simulink model "Tank_Backsteping_Adaptative_TIF"  (R2025b)
settings: Solver=ode45  StartTime=0.0  StopTime=250  RelTol=1e-3
model workspace (MAT data in the model file):
  Vp = Simulink.Parameter
  Vp.Complexity = 'real'
  Vp.Dimensions = [0 0]
  Vp.DataType = 'auto'
settings Model: Creator=juerg
settings DataIOCC: ReturnWorkspaceOutputs=off

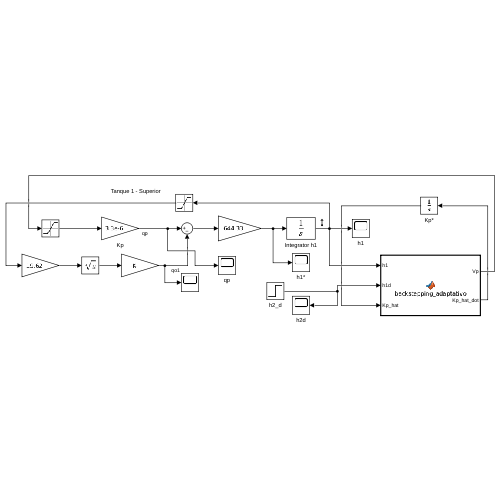
[thumbnail: Simulink's stored preview of the top-level diagram]
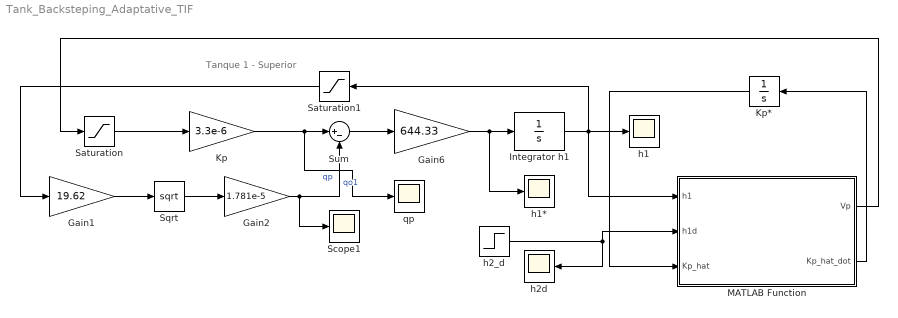
== system Tank_Backsteping_Adaptative_TIF ==
  note: Tanque 1 - Superior
  Gain1 : Gain  Gain=19.62
  Gain2 : Gain  Gain=1.781e-5
  Gain6 : Gain  Gain=644.33
  Integrator h1 : Integrator
  Kp : Gain  Gain=3.3e-6
  Kp* : Integrator  InitialCondition=6.82e-6
  MATLAB Function : MATLAB Function  TreatAsAtomicUnit=on
  Saturation : Saturate  UpperLimit=10  LowerLimit=0
  Saturation1 : Saturate  UpperLimit=Inf  LowerLimit=0
  Scope1 : Scope
      settings: ActiveDisplayYMinimum=-1  ActiveDisplayYMaximum=1  DataLoggingVariableName=ScopeData5
  Sqrt : Sqrt
  Sum : Sum  Inputs=|+-
  h1 : Scope
      settings: ActiveDisplayYMinimum=-0.0933782689070276  ActiveDisplayYMaximum=0.84040442016324857
  h1* : Scope
      settings: ActiveDisplayYMinimum=-0.0060808643749999981  ActiveDisplayYMaximum=0.054727779375  DataLoggingVariableName=ScopeData2
  h2_d : Step  Time=0.1  After=0.75  SampleTime=0
  h2d : Scope
      settings: ActiveDisplayYMinimum=-1  ActiveDisplayYMaximum=1  DataLoggingVariableName=ScopeData7
  qp : Scope
      settings: ActiveDisplayYMinimum=-1  ActiveDisplayYMaximum=1  DataLoggingVariableName=ScopeData4
  wires:
  Gain1/1 -> Sqrt/1
  Sqrt/1 -> Gain2/1
  Kp/1 -> qp/1, Sum/1  "qp"
  Gain2/1 -> Scope1/1, Sum/2  "qo1"
  Sum/1 -> Gain6/1
  Gain6/1 -> h1*/1, Integrator h1/1
  Integrator h1/1 -> MATLAB Function/1(h1), h1/1, Saturation1/1
  Saturation/1 -> Kp/1
  Saturation1/1 -> Gain1/1
  MATLAB Function/1(Vp) -> Saturation/1
  MATLAB Function/2(Kp_hat_dot) -> Kp*/1
  Kp*/1 -> MATLAB Function/3(Kp_hat)
  h2_d/1 -> MATLAB Function/2(h1d), h2d/1

== matlab function Tank_Backsteping_Adaptative_TIF/MATLAB Function ==
  data: h1 input; Vp output; h1d input; Kp_hat input; Kp_hat_dot output
function [Vp, Kp_hat_dot] = backstepping_adaptativo(h1, h1d, Kp_hat)
% Control backstepping adaptativo para UN SOLO tanque
% Entradas:
%   h1       -> nivel actual del tanque [m]
%   h1d      -> nivel deseado (referencia) [m]
%   Kp_hat   -> estimación actual de la ganancia de la bomba
% Salidas:
%   Vp          -> voltaje de control a la bomba [V]
%   Kp_hat_dot  -> derivada de la estimación Kp_hat

% --- 1) Parámetros del proceso ---
A1  = 1/644.33;        % [m^2]  área efectiva del tanque
Cv1 = 1.781e-5;        % [m^3/s/√m] coef. descarga orificio
c1  = 150;             % ganancia de estabilización (>0)
Gamma = 100.0;         % ganancia de adaptación (>0)

% --- 2) Error de seguimiento ---
z1 = h1 - h1d;

% --- 3) Ley de control (backstepping) ---
% Dinámica: A1 * dh1/dt = Kp*Vp - Cv1*sqrt(h1)
% Objetivo: dh1/dt = -c1*z1  (referencia constante)
% Control usando Kp_hat:
Vp_term = A1 * (-c1 * z1) + Cv1 * sqrt(h1);
Vp = Vp_term / max(Kp_hat, 1e-7);     % evita división por cero

% Saturación de actuador (0–10 V)
Vp = min(max(Vp, 0.0), 10.0);

% --- 4) Ley de adaptación de Kp ---
% Misma estructura que tenías: proporcional a error*entrada
Kp_hat_dot = Gamma * z1 * Vp;

% (Opcional) proyección para mantener Kp_hat físico, p. ej.:
% Kp_min = 1e-7; Kp_max = 5e-5;
% if Kp_hat <= Kp_min && Kp_hat_dot < 0, Kp_hat_dot = 0; end
% if Kp_hat >= Kp_max && Kp_hat_dot > 0, Kp_hat_dot = 0; end

end
